simulink model "QR2Dsim"  (R2013b)
settings: Solver=ode3  StartTime=0.0  StopTime=Tend_sim  FixedStep=.01  RelTol=1e-3
values from neighbouring files (symbols this model uses):
  b = 0.1    [QR2Drunfile.m]
  ctauf = 8.004e-3    (= 0.008004)    [QR2Drunfile.m]
  d = 0.1    [QR2Drunfile.m]
  DeltaR = [0.2; -0.1; 0.02]    [QR2Drunfile.m]
  Deltax = [-0.5; 0.2; 1]    [QR2Drunfile.m]
  dxL0 = 0    [QR2Drunfile.m]
  dyL0 = 0    [QR2Drunfile.m]
  dzL0 = 0    [QR2Drunfile.m]
  e3 = [0;0;1]    [QR2Drunfile.m]
  fc = (mQ+mL)*g    (= 44.5374)    [QR2Drunfile.m]
  fsat = [-1000 1000]    [QR2Drunfile.m]
  g = 9.81    [QR2Drunfile.m]
  I = diag([Ixx Iyy Izz])    [QR2Drunfile.m]
  Ir = 0.5    [QR2Drunfile.m]
  Ixx = 0.0820    (= 0.082)    [QR2Drunfile.m]
  Iyy = 0    [QR2Drunfile.m]
  Izz = 0    [QR2Drunfile.m]
  kdL = 1.4    [QR2Drunfile.m]
  kdQ = 5.6*mQ*.75    (= 18.228)    [QR2Drunfile.m]
  kdxL = 1    [QR2Drunfile.m]
  kOmega = kOmega_phi*eye(3)    [QR2Drunfile.m]
  kpL = 1.2    [QR2Drunfile.m]
  kpQ = 16*mQ    (= 69.44)    [QR2Drunfile.m]
  kpxL = 5    [QR2Drunfile.m]
  kR = kR_phi*eye(3)    [QR2Drunfile.m]
  l = 0.315    [QR2Drunfile.m]
  lL = 0.4    [QR2Drunfile.m]
  mL = 0.2    [QR2Drunfile.m]
  mode = 2    [QR2Drunfile.m]
  mQ = 4.34    [QR2Drunfile.m]
  omega0 = [0;0;0]    [QR2Drunfile.m]
  phiL0 = deg2rad(190)    [QR2Drunfile.m]
  phiLd = 0    [QR2Drunfile.m]
  phiQ0 = deg2rad(0)    [QR2Drunfile.m]
  phiQd = 0    [QR2Drunfile.m]
  pL0 = 0    [QR2Drunfile.m]
  pQ0 = 0    [QR2Drunfile.m]
  psiL0 = 0    [QR2Drunfile.m]
  psiQ0 = 0    [QR2Drunfile.m]
  qL0 = 0    [QR2Drunfile.m]
  qQ0 = 0    [QR2Drunfile.m]
  qvec0 = [0; sin(phiL0); cos(phiL0)]    [QR2Drunfile.m]
  Rinit = Rx    [QR2Drunfile.m]
  rL0 = 0    [QR2Drunfile.m]
  rQ0 = 0    [QR2Drunfile.m]
  thetaL0 = 0    [QR2Drunfile.m]
  thetaQ0 = 0    [QR2Drunfile.m]
  xLd = [0; 0; 0]    [QR2Drunfile.m]
undefined symbols (not defined in the file or in its folder): dx0, dy0, dz0, kv, kx, m, p0, q0, r0, x0, y0, z0
libraries: simulink_extras x10, vrlib x9, dspmathops x2
(part 1 of 2)
settings Model: Creator=Nam  LastModifiedBy=Nam
settings DataIOCC: SaveFormat=StructureWithTime
settings DebuggingCC: SolverPrmCheckMsg=none

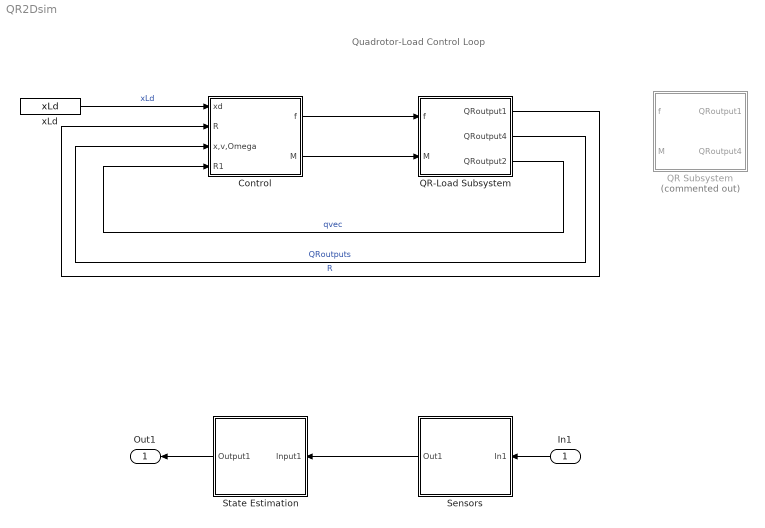
== system QR2Dsim ==
  note: Quadrotor-Load Control Loop
  In1 : Inport
  Control : Subsystem
  QR Subsystem : Subsystem  Commented=on
      mask Display: image('bebop.png')
  QR-Load Subsystem : Subsystem
  Sensors : Subsystem
      mask Display: image('optitrack.jpg')
  State Estimation : Subsystem
  xLd : Constant  Value=xLd  VectorParams1D=off
  Out1 : Outport
  wires:
  Sensors/1(Out1) -> State Estimation/1(Input1)
  State Estimation/1(Output1) -> Out1/1
  In1/1 -> Sensors/1(In1)
  QR-Load Subsystem/1(QRoutput1) -> Control/2(R)  "R"
  QR-Load Subsystem/2(QRoutput4) -> Control/3(x,v,Omega)  "QRoutputs"
  xLd/1 -> Control/1(xd)  "xLd"
  Control/1(f) -> QR-Load Subsystem/1(f)
  Control/2(M) -> QR-Load Subsystem/2(M)
  QR-Load Subsystem/3(QRoutput2) -> Control/4(R1)  "qvec"

== system QR2Dsim/Control ==
  note: Control
  xd : Inport
  R : Inport  Port=2
  x,v,Omega : Inport  Port=3
  R1 : Inport  Port=4
  QRL Load Attitude Controller : Subsystem
  QRL Load Position Controller : Subsystem
  QRL QR Attitude Controller : Subsystem
  Saturation : Saturate  UpperLimit=fsat(2)  LowerLimit=fsat(1)
  Terminator : Terminator
  f : Outport
  M : Outport  Port=2
  wires:
  R/1 -> QRL Load Position Controller/3(R1), QRL Load Attitude Controller/4(R), QRL QR Attitude Controller/3(R)
  x,v,Omega/1 -> QRL Load Attitude Controller/3(QROutput), QRL QR Attitude Controller/2(Omega), QRL Load Position Controller/2(QROutput1)
  Saturation/1 -> f/1  "f"
  xd/1 -> QRL Load Position Controller/1(xdes)
  QRL Load Position Controller/1(f) -> QRL Load Attitude Controller/1(xdes2), Saturation/1
  QRL QR Attitude Controller/1(M) -> M/1  "M"
  R1/1 -> Terminator/1  "qvec"
  QRL Load Attitude Controller/1(b3d1) -> QRL QR Attitude Controller/1(b1d)  "phiQc"
  QRL Load Position Controller/2(b3d1) -> QRL Load Attitude Controller/2(xdes1)

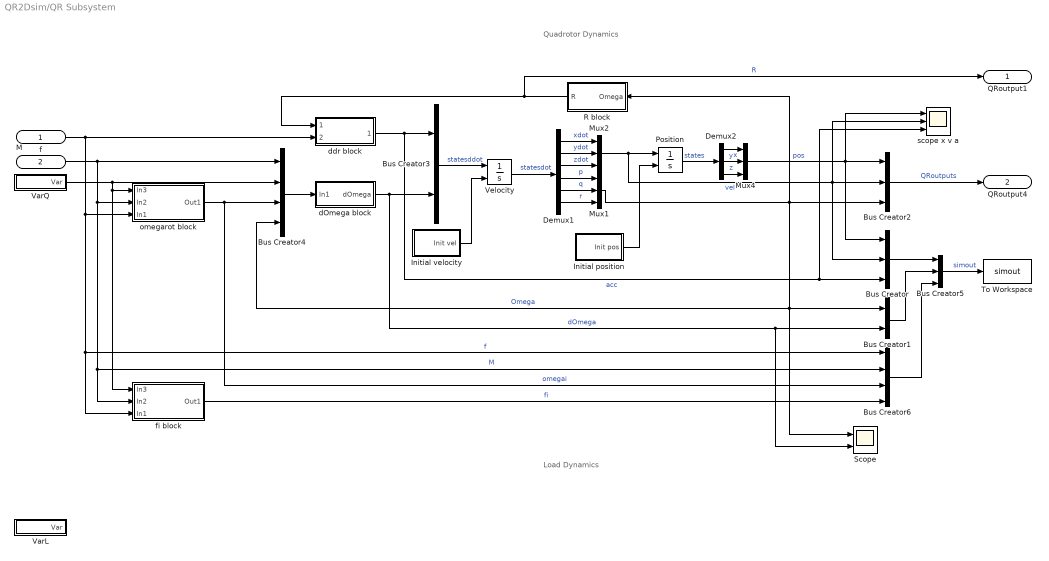
== system QR2Dsim/QR Subsystem ==
  note: Quadrotor Dynamics
  note: Load Dynamics
  f : Inport
  M : Inport  Port=2  PortDimensions=[3 1]
  Bus Creator : BusCreator  Inputs=3
  Bus Creator1 : BusCreator  Inputs=2
  Bus Creator2 : BusCreator  Inputs=3
  Bus Creator3 : BusCreator  Inputs=2
  Bus Creator4 : BusCreator
  Bus Creator5 : BusCreator  Inputs=3
  Bus Creator6 : BusCreator
  Demux1 : Demux  Outputs=6
  Demux2 : Demux  Outputs=3
  Initial position : Subsystem
  Initial velocity : Subsystem
  Mux1 : Mux  Inputs=3
  Mux2 : Mux  Inputs=3
  Mux4 : Mux  Inputs=3
  Position : Integrator  InitialConditionSource=external  ContinuousStateAttributes='position'
  R block : Subsystem
      mask Display: disp('R\prime = R \Omega_{\times}','texmode','on')
  Scope : Scope  NumInputPorts=2
      settings: ShowLegends=on  YMin=-5~-5  YMax=5~5  SaveName=ScopeData21
  To Workspace : ToWorkspace  VariableName=simout  SampleTime=-1  SaveFormat=Structure With Time
  VarL : Subsystem
  VarQ : Subsystem
  Velocity : Integrator  InitialConditionSource=external  ContinuousStateAttributes='velocity'
  dOmega block : Subsystem
      mask Display: disp('[p\prime; q\prime; r\prime]','texmode','on')
  ddr block : Subsystem
      mask Display: disp('[x\prime\prime; y\prime\prime; z\prime\prime]','texmode','on')
  fi block : Subsystem
      mask Display: disp('(f,M) \rightarrow f_i','texmode','on')
  omegarot block : Subsystem
      mask Display: disp('(f,M) \rightarrow \omega_i','texmode','on')
  scope x v a : Scope  NumInputPorts=3
      settings: ShowLegends=on  YMin=-10000~-500~0  YMax=180000~9000~225  SaveName=ScopeData12
  QRoutput1 : Outport
  QRoutput4 : Outport  Port=2
  wires:
  Velocity/1 -> Demux1/1  "statesdot"
  Position/1 -> Demux2/1  "states"
  ddr block/1(rddotOutput) -> Bus Creator3/1, Bus Creator/3, scope x v a/3  "acc"
  Bus Creator3/1 -> Velocity/1  "statesddot"
  dOmega block/1(dOmega) -> Bus Creator3/2, Bus Creator1/2, Scope/2  "dOmega"
  Bus Creator4/1 -> dOmega block/1(In1)
  Demux1/4 -> Mux1/1  "p"
  Demux1/5 -> Mux1/2  "q"
  Demux1/6 -> Mux1/3  "r"
  Demux1/2 -> Mux2/2  "ydot"
  Demux1/1 -> Mux2/1  "xdot"
  Demux1/3 -> Mux2/3  "zdot"
  Demux2/2 -> Mux4/2  "y"
  Demux2/1 -> Mux4/1  "x"
  Demux2/3 -> Mux4/3  "z"
  Mux4/1 -> scope x v a/1, Bus Creator/1, Bus Creator2/1  "pos"
  omegarot block/1(Out1) -> Bus Creator6/3, Bus Creator4/3  "omegai"
  Bus Creator/1 -> Bus Creator5/1
  Bus Creator1/1 -> Bus Creator5/2
  Bus Creator5/1 -> To Workspace/1  "simout"
  Mux1/1 -> Bus Creator2/3, R block/1(Omega), Bus Creator1/1, Scope/1, Bus Creator4/4  "Omega"
  Bus Creator2/1 -> QRoutput4/1  "QRoutputs"
  f/1 -> fi block/3(In1), Bus Creator6/1, omegarot block/3(In1), ddr block/2(R,f,m,g)  "f"
  VarQ/1(Var) -> fi block/1(In3), omegarot block/1(In3), Bus Creator4/2
  M/1 -> Bus Creator6/2, fi block/2(In2), omegarot block/2(In2), Bus Creator4/1  "M"
  Mux2/1 -> Position/1, scope x v a/2, Bus Creator/2, Bus Creator2/2  "vel"
  R block/1(R) -> ddr block/1(R,f,m,g1), QRoutput1/1  "R"
  Initial velocity/1(Init vel) -> Velocity/2
  Initial position/1(Init pos) -> Position/2
  fi block/1(Out1) -> Bus Creator6/4  "fi"
  Bus Creator6/1 -> Bus Creator5/3

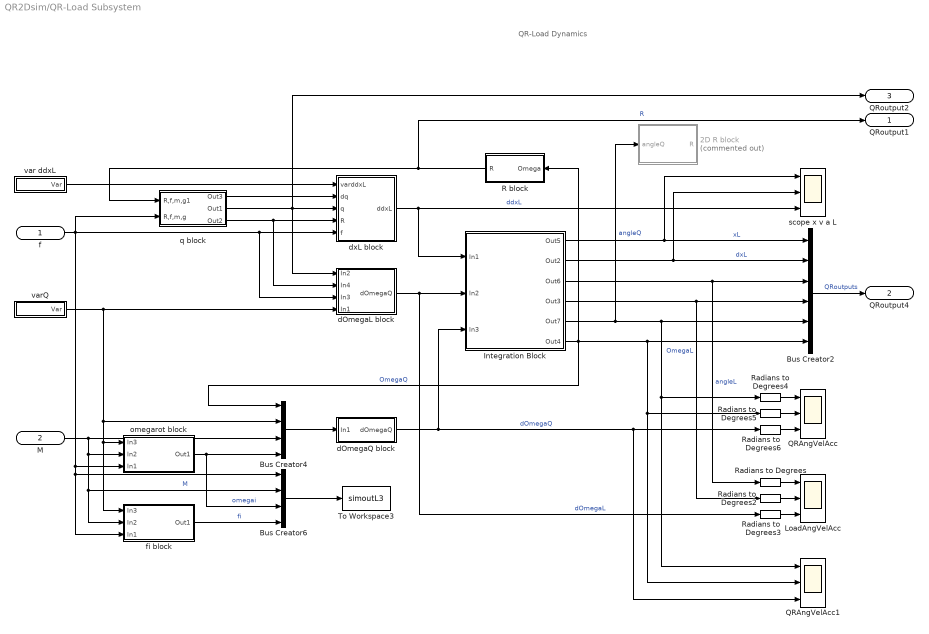
== system QR2Dsim/QR-Load Subsystem ==
  note: QR-Load Dynamics
  f : Inport
  M : Inport  Port=2  PortDimensions=3
  2D R block : MATLAB Function  Commented=on  TreatAsAtomicUnit=on
  Bus Creator2 : BusCreator  Inputs=6
  Bus Creator4 : BusCreator
  Bus Creator6 : BusCreator
  Integration Block : Subsystem
  LoadAngVelAcc : Scope  NumInputPorts=3
      settings: ShowLegends=on  YMin=-5~-5~-5  YMax=5~5~5  SaveName=ScopeData4
  QRAngVelAcc : Scope  NumInputPorts=3
      settings: ShowLegends=on  YMin=-5~-5~-5  YMax=5~5~5  SaveName=ScopeData3
  QRAngVelAcc1 : Scope  NumInputPorts=3
      settings: ShowLegends=on  YMin=-5~-5~-5  YMax=5~5~5  SaveName=ScopeData15
  R block : Subsystem
      mask Display: disp('R\prime = R \Omega_{\times}','texmode','on')
  Radians to Degrees{,2..6} (6 alike) : simulink_extras/Transformations/Radians to Degrees
  To Workspace3 : ToWorkspace  VariableName=simoutL3  SampleTime=-1  SaveFormat=Structure With Time
  dOmegaL block : Subsystem
  dOmegaQ block : Subsystem
  dxL block : MATLAB Function  TreatAsAtomicUnit=on
  fi block : Subsystem
      mask Display: disp('(f,M) \rightarrow f_i','texmode','on')
  omegarot block : Subsystem
      mask Display: disp('(f,M) \rightarrow \omega_i','texmode','on')
  q block : Subsystem
  scope x v a L : Scope  NumInputPorts=3
      settings: ShowLegends=on  YMin=-10000~-500~0  YMax=180000~9000~225  SaveName=ScopeData12
  var ddxL : Subsystem
  varQ : Subsystem
  QRoutput1 : Outport
  QRoutput4 : Outport  Port=2
  QRoutput2 : Outport  Port=3
  wires:
  dxL block/1(ddxL) -> scope x v a L/3, Integration Block/1(In1)  "ddxL"
  dOmegaQ block/1(dOmegaQ) -> Integration Block/3(In3), Radians to Degrees6/1, QRAngVelAcc1/3  "dOmegaQ"
  Bus Creator4/1 -> dOmegaQ block/1(In1)
  omegarot block/1(Out1) -> Bus Creator6/3, Bus Creator4/4  "omegai"
  Bus Creator2/1 -> QRoutput4/1  "QRoutputs"
  f/1 -> q block/2(R,f,m,g), dxL block/5(f), dOmegaL block/3(In3), omegarot block/3(In1), Bus Creator6/1, fi block/3(In1)
  M/1 -> fi block/2(In2), Bus Creator6/2, omegarot block/2(In2), Bus Creator4/3  "M"
  fi block/1(Out1) -> Bus Creator6/4  "fi"
  var ddxL/1(Var) -> dxL block/1(varddxL)
  q block/2(Out1) -> dxL block/3(q), QRoutput2/1, dOmegaL block/1(In2)
  q block/3(Out2) -> dxL block/4(R), dOmegaL block/2(In4)
  q block/1(Out3) -> dxL block/2(dq)
  Integration Block/5(Out7) -> Radians to Degrees4/1, QRAngVelAcc1/1, Bus Creator2/5, 2D R block/1(angleQ)  "angleQ"
  Integration Block/2(Out2) -> scope x v a L/2, Bus Creator2/2  "dxL"
  Integration Block/4(Out3) -> Bus Creator2/4, Radians to Degrees2/1  "OmegaL"
  Integration Block/6(Out4) -> R block/1(Omega), Radians to Degrees5/1, QRAngVelAcc1/2, Bus Creator2/6, Bus Creator4/1  "OmegaQ"
  Integration Block/1(Out5) -> scope x v a L/1, Bus Creator2/1  "xL"
  dOmegaL block/1(dOmegaQ) -> Radians to Degrees3/1, Integration Block/2(In2)  "dOmegaL"
  varQ/1(Var) -> Bus Creator4/2, fi block/1(In3), omegarot block/1(In3), dOmegaL block/4(In1)
  Integration Block/3(Out6) -> Bus Creator2/3, Radians to Degrees/1  "angleL"
  Bus Creator6/1 -> To Workspace3/1
  Radians to Degrees/1 -> LoadAngVelAcc/1
  Radians to Degrees2/1 -> LoadAngVelAcc/2
  Radians to Degrees3/1 -> LoadAngVelAcc/3
  Radians to Degrees5/1 -> QRAngVelAcc/2
  Radians to Degrees4/1 -> QRAngVelAcc/1
  Radians to Degrees6/1 -> QRAngVelAcc/3
  R block/1(R) -> q block/1(R,f,m,g1), QRoutput1/1  "R"

== system QR2Dsim/Sensors ==
  In1 : Inport
  Out1 : Outport
  wires:
  In1/1 -> Out1/1

== system QR2Dsim/State Estimation ==
  Input1 : Inport
  Output1 : Outport
  wires:
  Input1/1 -> Output1/1

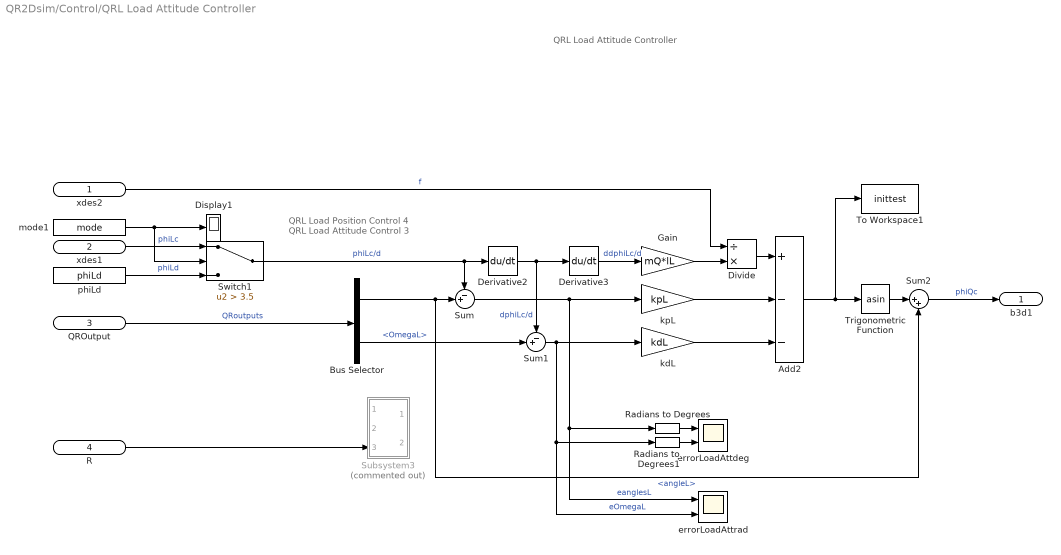
== system QR2Dsim/Control/QRL Load Attitude Controller ==
  note: QRL Load Attitude Controller
  note: QRL Load Position Control 4
      | QRL Load Attitude Control 3
  xdes2 : Inport
  xdes1 : Inport  Port=2
  QROutput : Inport  Port=3
  R : Inport  Port=4
  Add2 : Sum  Inputs=+--
  Bus Selector : BusSelector  OutputSignals=angleL,OmegaL
  Derivative2 : Derivative
  Derivative3 : Derivative
  Display1 : Display
  Divide : Product  Inputs=/*
  Gain : Gain  Gain=mQ*lL
  Radians to Degrees : simulink_extras/Transformations/Radians to Degrees
  Radians to Degrees1 : simulink_extras/Transformations/Radians to Degrees
  Subsystem3 : Subsystem  Commented=on
  Sum : Sum  Inputs=-+|
  Sum1 : Sum  Inputs=-+|
  Sum2 : Sum  Inputs=|++
  Switch1 : Switch  Criteria=u2 > Threshold  Threshold=3.5
  To Workspace1 : ToWorkspace  VariableName=inittest  SampleTime=-1  SaveFormat=Structure With Time
  Trigonometric Function : Trigonometry  Operator=asin
  errorLoadAttdeg : Scope  NumInputPorts=2
      settings: YMin=-5~-5  YMax=5~5  SaveName=ScopeData14
  errorLoadAttrad : Scope  NumInputPorts=2
      settings: YMin=-5~-5  YMax=5~5  SaveName=ScopeData26
  kdL : Gain  Gain=kdL
  kpL : Gain  Gain=kpL
  mode1 : Constant  Value=mode  VectorParams1D=off
  phiLd : Constant  Value=phiLd  VectorParams1D=off
  b3d1 : Outport
  wires:
  QROutput/1 -> Bus Selector/1  "QRoutputs"
  Sum/1 -> kpL/1, errorLoadAttrad/1, Radians to Degrees/1  "eanglesL"
  Sum1/1 -> kdL/1, errorLoadAttrad/2, Radians to Degrees1/1  "eOmegaL"
  kpL/1 -> Add2/2
  kdL/1 -> Add2/3
  Derivative2/1 -> Sum1/1, Derivative3/1  "dphiLc/d"
  Derivative3/1 -> Gain/1  "ddphiLc/d"
  Bus Selector/1 -> Sum2/2, Sum/2  "<angleL>"
  Bus Selector/2 -> Sum1/2  "<OmegaL>"
  Switch1/1 -> Derivative2/1, Sum/1  "phiLc/d"
  xdes1/1 -> Switch1/1  "phiLc"
  phiLd/1 -> Switch1/3  "phiLd"
  Sum2/1 -> b3d1/1  "phiQc"
  Gain/1 -> Divide/2
  Divide/1 -> Add2/1
  Add2/1 -> To Workspace1/1, Trigonometric Function/1
  Trigonometric Function/1 -> Sum2/1
  R/1 -> Subsystem3/3(In3)
  Radians to Degrees/1 -> errorLoadAttdeg/1
  Radians to Degrees1/1 -> errorLoadAttdeg/2
  xdes2/1 -> Divide/1  "f"
  mode1/1 -> Switch1/2, Display1/1

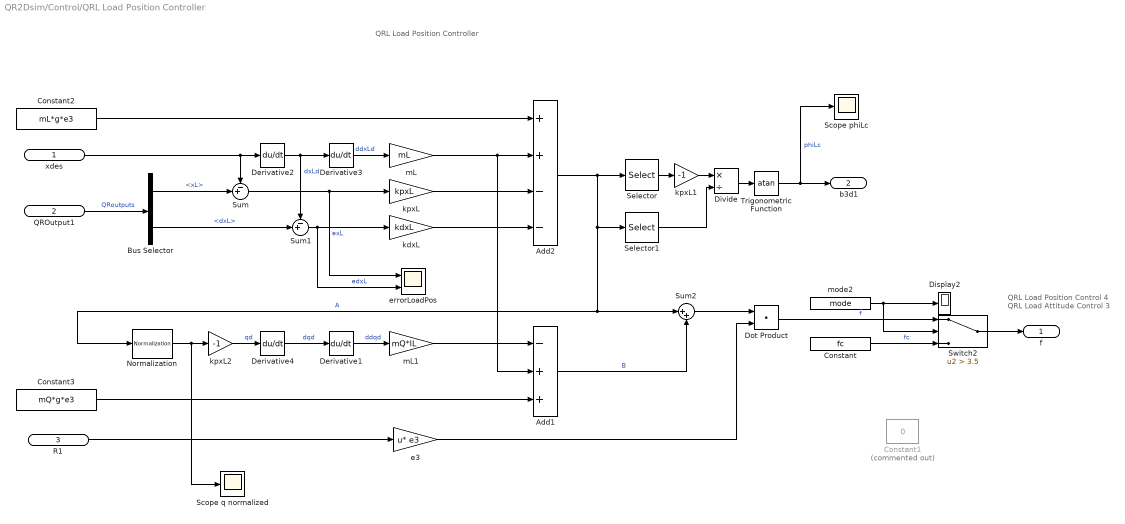
== system QR2Dsim/Control/QRL Load Position Controller ==
  note: QRL Load Position Controller
  note: QRL Load Position Control 4
      | QRL Load Attitude Control 3
  xdes : Inport
  QROutput1 : Inport  Port=2
  R1 : Inport  Port=3
  Add1 : Sum  Inputs=-++
  Add2 : Sum  Inputs=++--
  Bus Selector : BusSelector  OutputSignals=xL,dxL
  Constant : Constant  Value=fc
  Constant1 : Constant  Commented=on  Value=0
  Constant2 : Constant  Value=mL*g*e3
  Constant3 : Constant  Value=mQ*g*e3
  Derivative{1..4} (4 alike) : Derivative
  Display2 : Display
  Divide : Product  Inputs=*/
  Dot Product : DotProduct  InputSameDT=on  OutDataTypeStr=Inherit: Inherit via internal rule
  Normalization : dspmathops/Normalization  NormType=2-norm  Bias=1e-10  NormOver=Each column  ColComp=on  Dimension=1  outputDataTypeStr=Inherit: Same as product output  outputLastDataTypeStr=Inherit: Same as product output  outputMin=[]  outputMax=[]  accumDataTypeStr=Inherit: Same as product output  accumLastDataTypeStr=Inherit: Same as product output  roundingMode=Floor  overflowMode=off
  Scope phiLc : Scope
      settings: SaveName=ScopeData27
  Scope q normalized : Scope
      settings: SaveName=ScopeData29
  Selector : Selector  InputPortWidth=3  IndexOptions=Index vector (dialog)  Indices=2  OutputSizes=1
  Selector1 : Selector  InputPortWidth=3  IndexOptions=Index vector (dialog)  Indices=3  OutputSizes=1
  Sum : Sum  Inputs=-+|
  Sum1 : Sum  Inputs=-+|
  Sum2 : Sum  Inputs=|++
  Switch2 : Switch  Criteria=u2 > Threshold  Threshold=3.5
  Trigonometric Function : Trigonometry  Operator=atan
  e3 : Gain  Gain=e3  Multiplication=Matrix(u*K)
  errorLoadPos : Scope  NumInputPorts=2
      settings: YMin=-5~-5  YMax=5~5  SaveName=ScopeData28
  kdxL : Gain  Gain=kdxL
  kpxL : Gain  Gain=kpxL
  kpxL1 : Gain  Gain=-1
  kpxL2 : Gain  Gain=-1
  mL : Gain  Gain=mL
  mL1 : Gain  Gain=mQ*lL
  mode2 : Constant  Value=mode  VectorParams1D=off
  f : Outport
  b3d1 : Outport  Port=2
  wires:
  QROutput1/1 -> Bus Selector/1  "QRoutputs"
  Sum/1 -> kpxL/1, errorLoadPos/1  "exL"
  Sum1/1 -> kdxL/1, errorLoadPos/2  "edxL"
  kpxL/1 -> Add2/3
  kdxL/1 -> Add2/4
  Derivative2/1 -> Sum1/1, Derivative3/1  "dxLd"
  Derivative3/1 -> mL/1  "ddxLd"
  Bus Selector/1 -> Sum/2  "<xL>"
  Bus Selector/2 -> Sum1/2  "<dxL>"
  xdes/1 -> Derivative2/1, Sum/1
  mL/1 -> Add1/2, Add2/2
  Constant2/1 -> Add2/1
  Add2/1 -> Normalization/1, Sum2/1, Selector1/1, Selector/1  "A"
  R1/1 -> e3/1
  e3/1 -> Dot Product/2
  Add1/1 -> Sum2/2  "B"
  Sum2/1 -> Dot Product/1
  Selector/1 -> kpxL1/1
  kpxL1/1 -> Divide/1
  Selector1/1 -> Divide/2
  Divide/1 -> Trigonometric Function/1
  Trigonometric Function/1 -> Scope phiLc/1, b3d1/1  "phiLc"
  Normalization/1 -> Scope q normalized/1, kpxL2/1
  kpxL2/1 -> Derivative4/1  "qd"
  Derivative4/1 -> Derivative1/1  "dqd"
  Derivative1/1 -> mL1/1  "ddqd"
  mL1/1 -> Add1/1
  Constant3/1 -> Add1/3
  Constant/1 -> Switch2/3  "fc"
  mode2/1 -> Switch2/2, Display2/1
  Switch2/1 -> f/1
  Dot Product/1 -> Switch2/1  "f"

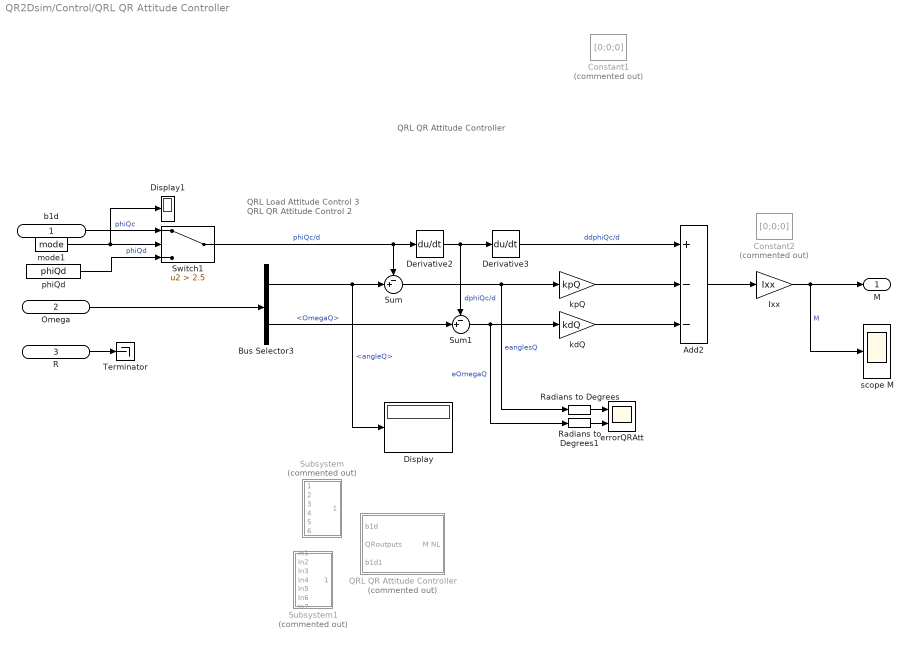
== system QR2Dsim/Control/QRL QR Attitude Controller ==
  note: QRL QR Attitude Controller
  note: QRL Load Attitude Control 3
      | QRL QR Attitude Control 2
  b1d : Inport
  Omega : Inport  Port=2
  R : Inport  Port=3
  Add2 : Sum  Inputs=+--
  Bus Selector3 : BusSelector  OutputSignals=angleQ,OmegaQ
  Constant1 : Constant  Commented=on  Value=[0;0;0]
  Constant2 : Constant  Commented=on  Value=[0;0;0]
  Derivative2 : Derivative
  Derivative3 : Derivative
  Display : Display
  Display1 : Display
  Ixx : Gain  Gain=Ixx
  QRL QR Attitude Controller : Subsystem  Commented=on
  Radians to Degrees : simulink_extras/Transformations/Radians to Degrees
  Radians to Degrees1 : simulink_extras/Transformations/Radians to Degrees
  Subsystem : Subsystem  Commented=on
  Subsystem1 : Subsystem  Commented=on
  Sum : Sum  Inputs=-+|
  Sum1 : Sum  Inputs=-+|
  Switch1 : Switch  Criteria=u2 > Threshold  Threshold=2.5
  Terminator : Terminator
  errorQRAtt : Scope  NumInputPorts=2
      settings: YMin=-5~-5  YMax=5~5  SaveName=ScopeData6
  kdQ : Gain  Gain=kdQ
  kpQ : Gain  Gain=kpQ
  mode1 : Constant  Value=mode  VectorParams1D=off
  phiQd : Constant  Value=phiQd  VectorParams1D=off
  scope M : Scope
      settings: ShowLegends=on  SaveName=ScopeData19
  M : Outport  PortDimensions=3
  wires:
  mode1/1 -> Display1/1, Switch1/2
  b1d/1 -> Switch1/1  "phiQc"
  phiQd/1 -> Switch1/3  "phiQd"
  Omega/1 -> Bus Selector3/1
  Sum/1 -> Radians to Degrees/1, kpQ/1  "eanglesQ"
  Sum1/1 -> Radians to Degrees1/1, kdQ/1  "eOmegaQ"
  Ixx/1 -> scope M/1, M/1  "M"
  kpQ/1 -> Add2/2
  kdQ/1 -> Add2/3
  Add2/1 -> Ixx/1
  Switch1/1 -> Derivative2/1, Sum/1  "phiQc/d"
  Derivative2/1 -> Sum1/1, Derivative3/1  "dphiQc/d"
  Derivative3/1 -> Add2/1  "ddphiQc/d"
  Bus Selector3/1 -> Sum/2, Display/1  "<angleQ>"
  Bus Selector3/2 -> Sum1/2  "<OmegaQ>"
  R/1 -> Terminator/1
  Radians to Degrees/1 -> errorQRAtt/1
  Radians to Degrees1/1 -> errorQRAtt/2

== system QR2Dsim/QR Subsystem/Initial position ==
  Bus Creator2 : BusCreator  Inputs=3
  x0 : Constant  Value=x0
  y0 : Constant  Value=y0
  z0 : Constant  Value=z0
  Init pos : Outport
  wires:
  y0/1 -> Bus Creator2/2  "y0"
  x0/1 -> Bus Creator2/1  "x0"
  z0/1 -> Bus Creator2/3  "z0"
  Bus Creator2/1 -> Init pos/1  "Init pos"

== system QR2Dsim/QR Subsystem/Initial velocity ==
  Bus Creator1 : BusCreator  Inputs=6
  dx0 : Constant  Value=dx0
  dy0 : Constant  Value=dy0
  dz0 : Constant  Value=dz0
  p0 : Constant  Value=p0
  q0 : Constant  Value=q0
  r0 : Constant  Value=r0
  Init vel : Outport
  wires:
  p0/1 -> Bus Creator1/4  "p0"
  dx0/1 -> Bus Creator1/1  "dx0"
  dz0/1 -> Bus Creator1/3  "dz0"
  dy0/1 -> Bus Creator1/2  "dy0"
  q0/1 -> Bus Creator1/5  "q0"
  r0/1 -> Bus Creator1/6  "r0"
  Bus Creator1/1 -> Init vel/1  "Init vel"

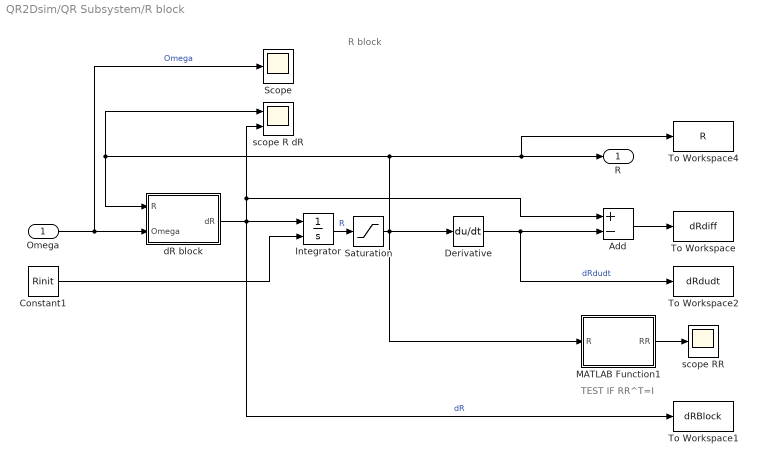
== system QR2Dsim/QR Subsystem/R block ==
  note: R block
  note: TEST IF RR^T=I
  Omega : Inport
  Add : Sum  Inputs=+-
  Constant1 : Constant  Value=Rinit
  Derivative : Derivative
  Integrator : Integrator  InitialConditionSource=external  ContinuousStateAttributes='R'
  MATLAB Function1 : MATLAB Function  TreatAsAtomicUnit=on
  Saturation : Saturate  UpperLimit=1  LowerLimit=-1
  Scope : Scope
      settings: ShowLegends=on  SaveName=ScopeData9
  To Workspace : ToWorkspace  VariableName=dRdiff  SampleTime=-1  SaveFormat=Structure With Time
  To Workspace1 : ToWorkspace  VariableName=dRBlock  SampleTime=-1  SaveFormat=Structure With Time
  To Workspace2 : ToWorkspace  VariableName=dRdudt  SampleTime=-1  SaveFormat=Structure With Time
  To Workspace4 : ToWorkspace  VariableName=R  SampleTime=-1  SaveFormat=Structure With Time
  dR block : MATLAB Function  TreatAsAtomicUnit=on
  scope R dR : Scope  NumInputPorts=2
      settings: ShowLegends=on  YMin=-1.2~-4e+19  YMax=1.2~4e+19  SaveName=ScopeData16
  scope RR : Scope
      settings: SaveName=ScopeData17
  R : Outport
  wires:
  Integrator/1 -> Saturation/1  "R"
  dR block/1(dR) -> scope R dR/2, Add/1, To Workspace1/1, Integrator/1  "dR"
  Omega/1 -> Scope/1, dR block/2(Omega)  "Omega"
  Derivative/1 -> Add/2, To Workspace2/1  "dRdudt"
  Add/1 -> To Workspace/1
  MATLAB Function1/1(RR) -> scope RR/1
  Constant1/1 -> Integrator/2
  Saturation/1 -> MATLAB Function1/1(R), Derivative/1, dR block/1(R), scope R dR/1, R/1, To Workspace4/1

== system QR2Dsim/QR Subsystem/VarL ==
  Bus Creator : BusCreator  Inputs=2
  Bus Creator1 : BusCreator  Inputs=2
  Cable length : Constant  Value=lL
  Gravity Constant : Constant  Value=g
  Mass Load : Constant  Value=mL
  Var : Outport
  wires:
  Gravity Constant/1 -> Bus Creator/2  "g"
  Bus Creator/1 -> Var/1  "varL"
  Mass Load/1 -> Bus Creator1/1  "mL"
  Cable length/1 -> Bus Creator1/2  "lL"
  Bus Creator1/1 -> Bus Creator/1  "sysvar"

== system QR2Dsim/QR Subsystem/VarQ ==
  Arm length : Constant  Value=l
  Bus Creator : BusCreator  Inputs=2
  Bus Creator1 : BusCreator  Inputs=7
  Drag Factor : Constant  Value=d
  Gravity Constant : Constant  Value=g
  Mass QR : Constant  Value=mQ
  QR Inertia : Constant  Value=diag([Ixx,Iyy,Izz])
  Rotor Inertia : Constant  Value=Ir
  Thrust Factor : Constant  Value=b
  ctauf : Constant  Value=ctauf
      mask Display: disp('c_{\tau f}','texmode','on')
  Var : Outport
  wires:
  Gravity Constant/1 -> Bus Creator/2  "g"
  Bus Creator/1 -> Var/1  "varQ"
  Mass QR/1 -> Bus Creator1/1  "m"
  Arm length/1 -> Bus Creator1/6  "l"
  Rotor Inertia/1 -> Bus Creator1/5  "Ir"
  QR Inertia/1 -> Bus Creator1/2  "I"
  Bus Creator1/1 -> Bus Creator/1  "sysvar"
  Thrust Factor/1 -> Bus Creator1/3  "b"
  Drag Factor/1 -> Bus Creator1/4  "d"
  ctauf/1 -> Bus Creator1/7  "ctauf"

== system QR2Dsim/QR Subsystem/dOmega block ==
  In1 : Inport
  Add : Sum  Inputs=-+
  Bus Selector : BusSelector  OutputSignals=Omega,varQ.sysvar.Ir,omegai,M
  DeltaR : Constant  Value=DeltaR
      mask Display: disp('\Delta_R','texmode','on')
  Gain : Gain  Gain=inv(I)  Multiplication=Matrix(K*u)
  Subsystem1 : Subsystem
      mask Display: disp('\Omega \times I\Omega','texmode','on')
  Subsystem2 : Subsystem
      mask Display: disp('\tau_G=\Sigma I_R(\omega \times e_3) \omega_i ','texmode','on')
  Terminator : Terminator
  Terminator1 : Terminator
  dOmega : Outport
  wires:
  In1/1 -> Bus Selector/1
  Bus Selector/1 -> Subsystem1/1(Omega), Subsystem2/1(In1)  "<Omega>"
  Bus Selector/2 -> Subsystem2/2(In2)  "<Ir>"
  Bus Selector/4 -> Add/2  "<M>"
  Subsystem2/1(Out1) -> Terminator/1
  Bus Selector/3 -> Subsystem2/3(In3)  "<omegai>"
  DeltaR/1 -> Terminator1/1  "DeltaR"
  Subsystem1/1(Out1) -> Add/1
  Add/1 -> Gain/1  "J*dOmega"
  Gain/1 -> dOmega/1

== system QR2Dsim/QR Subsystem/ddr block ==
  R,f,m,g1 : Inport
  R,f,m,g : Inport  Port=2
  Deltax : Constant  Value=Deltax
      mask Display: disp('\Delta_x','texmode','on')
  Gain : Gain  Gain=e3  Multiplication=Matrix(u*K)
  Gain1 : Gain  Gain=1/m
  Product : Product
  Sum : Sum  Inputs=|-+
  Terminator : Terminator
  mge3 : Constant  Value=m*g*e3
  rddotOutput : Outport
  wires:
  R,f,m,g1/1 -> Gain/1  "R"
  R,f,m,g/1 -> Product/2  "f"
  Gain/1 -> Product/1
  Product/1 -> Sum/1
  mge3/1 -> Sum/2  "m"
  Sum/1 -> Gain1/1
  Gain1/1 -> rddotOutput/1  "a"
  Deltax/1 -> Terminator/1  "Deltax"

== system QR2Dsim/QR Subsystem/fi block ==
  In3 : Inport
  In2 : Inport  Port=2
  In1 : Inport  Port=3
  Bus Selector2 : BusSelector  OutputSignals=sysvar.l,sysvar.ctauf  OutputAsBus=on
  Saturation : Saturate  UpperLimit=inf  LowerLimit=-inf  ZeroCross=off
  fcnf : MATLAB Function  TreatAsAtomicUnit=on
  Out1 : Outport
  wires:
  In3/1 -> Bus Selector2/1
  In1/1 -> fcnf/3(f)  "f"
  In2/1 -> fcnf/2(M)  "M"
  Bus Selector2/1 -> fcnf/1(var)  "var"
  fcnf/1(fi) -> Saturation/1
  Saturation/1 -> Out1/1  "fi"

== system QR2Dsim/QR Subsystem/omegarot block ==
  In3 : Inport
  In2 : Inport  Port=2
  In1 : Inport  Port=3
  Bus Selector2 : BusSelector  OutputSignals=sysvar.b,sysvar.d,sysvar.l  OutputAsBus=on
  Saturation : Saturate  UpperLimit=inf  LowerLimit=0  ZeroCross=off
  Sqrt : Sqrt  SaturateOnIntegerOverflow=on
  fcnomega : MATLAB Function  TreatAsAtomicUnit=on
  Out1 : Outport
  wires:
  In3/1 -> Bus Selector2/1
  In1/1 -> fcnomega/3(f)  "f"
  In2/1 -> fcnomega/2(M)  "M"
  Bus Selector2/1 -> fcnomega/1(var)  "var"
  Sqrt/1 -> Out1/1  "omegai"
  Saturation/1 -> Sqrt/1
  fcnomega/1(omegai) -> Saturation/1  "omegai^2"

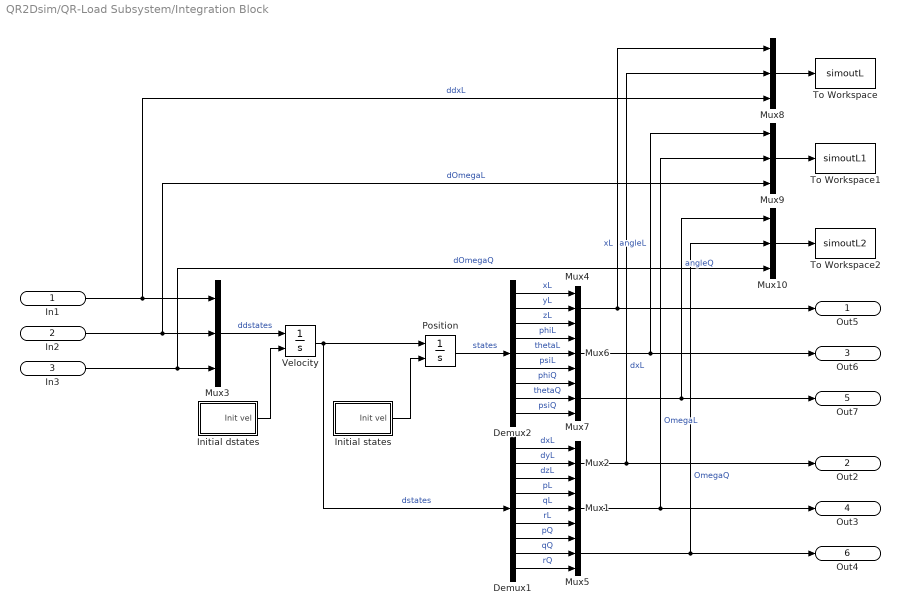
== system QR2Dsim/QR-Load Subsystem/Integration Block ==
  In1 : Inport
  In2 : Inport  Port=2
  In3 : Inport  Port=3
  Demux1 : Demux  Outputs=9
  Demux2 : Demux  Outputs=9
  Initial dstates : Subsystem
  Initial states : Subsystem
  Mux{1..10} (10 alike) : Mux  Inputs=3
  Position : Integrator  InitialConditionSource=external  ContinuousStateAttributes='position'
  To Workspace : ToWorkspace  VariableName=simoutL  SampleTime=-1  SaveFormat=Structure With Time
  To Workspace1 : ToWorkspace  VariableName=simoutL1  SampleTime=-1  SaveFormat=Structure With Time
  To Workspace2 : ToWorkspace  VariableName=simoutL2  SampleTime=-1  SaveFormat=Structure With Time
  Velocity : Integrator  InitialConditionSource=external  ContinuousStateAttributes='velocity'
  Out5 : Outport
  Out2 : Outport  Port=2
  Out6 : Outport  Port=3
  Out3 : Outport  Port=4
  Out7 : Outport  Port=5
  Out4 : Outport  Port=6
  wires:
  In1/1 -> Mux8/3, Mux3/1  "ddxL"
  Demux1/4 -> Mux1/1  "pL"
  Demux1/5 -> Mux1/2  "qL"
  Demux1/6 -> Mux1/3  "rL"
  Demux1/2 -> Mux2/2  "dyL"
  Demux1/1 -> Mux2/1  "dxL"
  Demux1/3 -> Mux2/3  "dzL"
  Demux1/8 -> Mux5/2  "qQ"
  Demux1/9 -> Mux5/3  "rQ"
  Demux1/7 -> Mux5/1  "pQ"
  Mux3/1 -> Velocity/1  "ddstates"
  Initial dstates/1(Init vel) -> Velocity/2
  Position/1 -> Demux2/1  "states"
  Demux2/2 -> Mux4/2  "yL"
  Demux2/1 -> Mux4/1  "xL"
  Demux2/3 -> Mux4/3  "zL"
  Initial states/1(Init vel) -> Position/2
  Demux2/4 -> Mux6/1  "phiL"
  Demux2/5 -> Mux6/2  "thetaL"
  Demux2/6 -> Mux6/3  "psiL"
  Demux2/9 -> Mux7/3  "psiQ"
  Demux2/8 -> Mux7/2  "thetaQ"
  Demux2/7 -> Mux7/1  "phiQ"
  Velocity/1 -> Position/1, Demux1/1  "dstates"
  Mux2/1 -> Mux8/2, Out2/1  "dxL"
  Mux4/1 -> Mux8/1, Out5/1  "xL"
  Mux1/1 -> Mux9/2, Out3/1  "OmegaL"
  In2/1 -> Mux9/3, Mux3/2  "dOmegaL"
  Mux6/1 -> Mux9/1, Out6/1  "angleL"
  In3/1 -> Mux10/3, Mux3/3  "dOmegaQ"
  Mux7/1 -> Mux10/1, Out7/1  "angleQ"
  Mux5/1 -> Mux10/2, Out4/1  "OmegaQ"
  Mux8/1 -> To Workspace/1
  Mux9/1 -> To Workspace1/1
  Mux10/1 -> To Workspace2/1

== system QR2Dsim/QR-Load Subsystem/R block ==
  note: R block
  Omega : Inport
  Constant1 : Constant  Value=Rinit
  Integrator : Integrator  InitialConditionSource=external  ContinuousStateAttributes='R'
  Saturation : Saturate  UpperLimit=1  LowerLimit=-1
  To Workspace4 : ToWorkspace  VariableName=R  SampleTime=-1  SaveFormat=Structure With Time
  dR block : MATLAB Function  TreatAsAtomicUnit=on
  R : Outport
  wires:
  Integrator/1 -> Saturation/1  "R"
  dR block/1(dR) -> Integrator/1
  Omega/1 -> dR block/2(Omega)
  Constant1/1 -> Integrator/2
  Saturation/1 -> dR block/1(R), To Workspace4/1, R/1  "R"

== system QR2Dsim/QR-Load Subsystem/dOmegaL block ==
  note: dOmegaL block
  In2 : Inport
  In4 : Inport  Port=2
  In3 : Inport  Port=3
  In1 : Inport  Port=4
  Bus Selector : BusSelector  OutputSignals=sysvar.m,sysvar.lL
  Cross Product : vrlib/Utilities/Cross Product
  Divide : Product  Inputs=*/
  Gain : Gain  Gain=-1
  Gain1 : Gain  Gain=e3  Multiplication=Matrix(u*K)
  Product1 : Product
  Product2 : Product
  dOmegaQ : Outport
  wires:
  In2/1 -> Gain/1  "q"
  In3/1 -> Product1/1  "f"
  In4/1 -> Gain1/1  "R"
  Gain/1 -> Cross Product/1
  Gain1/1 -> Product1/2  "Re3"
  Product1/1 -> Cross Product/2
  In1/1 -> Bus Selector/1  "varQ"
  Bus Selector/1 -> Product2/1  "<m>"
  Bus Selector/2 -> Product2/2  "<lL>"
  Cross Product/1 -> Divide/1
  Product2/1 -> Divide/2
  Divide/1 -> dOmegaQ/1  "dOmegaL"

== system QR2Dsim/QR-Load Subsystem/dOmegaQ block ==
  In1 : Inport
  Add : Sum  Inputs=-+
  Bus Selector : BusSelector  OutputSignals=OmegaQ,varQ.sysvar.Ir,omegai,M
  Gain1 : Gain  Gain=0
  Gain2 : Gain  Gain=inv(Ixx)
  Subsystem1 : Subsystem
      mask Display: disp('\Omega \times I\Omega','texmode','on')
  Subsystem2 : Subsystem
      mask Display: disp('\tau_G=\Sigma I_R(\omega \times e_3) \omega_i ','texmode','on')
  Terminator : Terminator
  dOmegaQ : Outport
  wires:
  In1/1 -> Bus Selector/1  "varQ"
  Bus Selector/1 -> Subsystem1/1(Omega), Subsystem2/1(In1)  "<OmegaQ>"
  Bus Selector/2 -> Subsystem2/2(In2)  "<Ir>"
  Subsystem2/1(Out1) -> Terminator/1
  Bus Selector/3 -> Subsystem2/3(In3)  "<omegai>"
  Subsystem1/1(Out1) -> Gain1/1
  Gain1/1 -> Add/1
  Add/1 -> Gain2/1  "J*dOmega"
  Bus Selector/4 -> Add/2  "<M>"
  Gain2/1 -> dOmegaQ/1  "dOmegaQ"

== system QR2Dsim/QR-Load Subsystem/fi block ==
  In3 : Inport
  In2 : Inport  Port=2
  In1 : Inport  Port=3
  Bus Selector2 : BusSelector  OutputSignals=sysvar.l,sysvar.ctauf  OutputAsBus=on
  Saturation : Saturate  UpperLimit=inf  LowerLimit=-inf  ZeroCross=off
  fcnf : MATLAB Function  TreatAsAtomicUnit=on
  Out1 : Outport
  wires:
  In3/1 -> Bus Selector2/1
  In1/1 -> fcnf/3(f)  "f"
  In2/1 -> fcnf/2(M)  "M"
  Bus Selector2/1 -> fcnf/1(var)  "var"
  fcnf/1(fi) -> Saturation/1
  Saturation/1 -> Out1/1  "fi"

== system QR2Dsim/QR-Load Subsystem/omegarot block ==
  In3 : Inport
  In2 : Inport  Port=2
  In1 : Inport  Port=3
  Bus Selector2 : BusSelector  OutputSignals=sysvar.b,sysvar.d,sysvar.l  OutputAsBus=on
  Saturation : Saturate  UpperLimit=inf  LowerLimit=0  ZeroCross=off
  Sqrt : Sqrt  SaturateOnIntegerOverflow=on
  fcnomega : MATLAB Function  TreatAsAtomicUnit=on
  Out1 : Outport
  wires:
  In3/1 -> Bus Selector2/1
  In1/1 -> fcnomega/3(f)  "f"
  In2/1 -> fcnomega/2(M)  "M"
  Bus Selector2/1 -> fcnomega/1(var)  "var"
  Sqrt/1 -> Out1/1  "omegai"
  Saturation/1 -> Sqrt/1
  fcnomega/1(omegai) -> Saturation/1  "omegai^2"

== system QR2Dsim/QR-Load Subsystem/q block ==
  note: q Block
  R,f,m,g1 : Inport
  R,f,m,g : Inport  Port=2
  1/(mQ*lL) : Gain  Gain=1/(mQ*lL)
  Cross Product : vrlib/Utilities/Cross Product
  Cross Product1 : vrlib/Utilities/Cross Product
  Gain : Gain  Gain=e3  Multiplication=Matrix(u*K)
  Gain1 : Gain  Gain=-1
  Integrator1 : Integrator  InitialCondition=qvec0  ContinuousStateAttributes='velocity'
  Integrator2 : Integrator  InitialCondition=omega0  ContinuousStateAttributes='velocity'
  Product : Product
  To Workspace1 : ToWorkspace  VariableName=qvec  SampleTime=-1  SaveFormat=Structure With Time
  Out3 : Outport
  Out1 : Outport  Port=2
  Out2 : Outport  Port=3
  wires:
  Cross Product/1 -> Integrator1/1, Out3/1  "dq"
  Integrator1/1 -> Out1/1, To Workspace1/1, Cross Product/2, Gain1/1  "q"
  Integrator2/1 -> Cross Product/1  "omega"
  R,f,m,g1/1 -> Gain/1, Out2/1  "R"
  Gain/1 -> Product/2  "Re3"
  Product/1 -> Cross Product1/2
  Gain1/1 -> Cross Product1/1
  Cross Product1/1 -> 1/(mQ*lL)/1
  1/(mQ*lL)/1 -> Integrator2/1  "domega"
  R,f,m,g/1 -> Product/1  "f"

== system QR2Dsim/QR-Load Subsystem/var ddxL ==
  Bus Creator1 : BusCreator
  Cable length : Constant  Value=lL
  Gravity Constant : Constant  Value=g
  Mass Load : Constant  Value=mL
  Mass QR : Constant  Value=mQ
  Var : Outport
  wires:
  Mass QR/1 -> Bus Creator1/1  "mQ"
  Cable length/1 -> Bus Creator1/4  "lL"
  Mass Load/1 -> Bus Creator1/3  "mL"
  Bus Creator1/1 -> Var/1  "varddxL"
  Gravity Constant/1 -> Bus Creator1/2  "g"

== system QR2Dsim/QR-Load Subsystem/varQ ==
  Arm length : Constant  Value=l
  Bus Creator : BusCreator  Inputs=2
  Bus Creator1 : BusCreator  Inputs=8
  Cable length : Constant  Value=lL
  Drag Factor : Constant  Value=d
  Gravity Constant : Constant  Value=g
  Mass QR : Constant  Value=mQ
  QR Inertia : Constant  Value=diag([Ixx,Iyy,Izz])
  Rotor Inertia : Constant  Value=Ir
  Thrust Factor : Constant  Value=b
  ctauf : Constant  Value=ctauf
      mask Display: disp('c_{\tau f}','texmode','on')
  Var : Outport
  wires:
  Gravity Constant/1 -> Bus Creator/2  "g"
  Bus Creator/1 -> Var/1  "varQ"
  Mass QR/1 -> Bus Creator1/1  "m"
  Arm length/1 -> Bus Creator1/6  "l"
  Rotor Inertia/1 -> Bus Creator1/5  "Ir"
  QR Inertia/1 -> Bus Creator1/2  "I"
  Bus Creator1/1 -> Bus Creator/1  "sysvar"
  Thrust Factor/1 -> Bus Creator1/3  "b"
  Drag Factor/1 -> Bus Creator1/4  "d"
  ctauf/1 -> Bus Creator1/7  "ctauf"
  Cable length/1 -> Bus Creator1/8  "lL"

== system QR2Dsim/Control/QRL Load Attitude Controller/Subsystem3 ==
  note: Attitude Controlled Flight Mode
  note: Position Controlled Flight Mode Lee2010c
  note: Attitude Control 1
      | Position Control 0
  In1 : Inport
  In2 : Inport  Port=2
  In3 : Inport  Port=3
  Display : Display  Commented=on
  Gain1 : Gain  Commented=on
  Gain5 : Gain  Commented=on
  Subsystem : Subsystem  Commented=on
  Subsystem1 : Subsystem  Commented=on
  Subsystem2 : Subsystem  Commented=on
  Switch : Switch  Commented=on  Criteria=u2 > Threshold  Threshold=0.5
  To Workspace : ToWorkspace  Commented=on  VariableName=Re3  SampleTime=-1  SaveFormat=Structure With Time
  "e3 " : Gain  Commented=on  Gain=e3  Multiplication=Matrix(u*K)
  mode : Constant  Commented=on  Value=mode  VectorParams1D=off
  scope fatt fpos1 : Scope  Commented=on  NumInputPorts=2
      settings: ShowLegends=on  YMin=-11000~-200  YMax=5000~150  SaveName=ScopeData25
  Out1 : Outport
  Out2 : Outport  Port=2
  wires:
  In3/1 -> "e3 "/1
  "e3 "/1 -> Subsystem/5(Re3), Subsystem2/5(Re3), To Workspace/1
  Subsystem/1(fatt) -> Gain5/1
  Gain5/1 -> Switch/1, scope fatt fpos1/1  "fatt"
  Subsystem2/2(fpos) -> Switch/3, scope fatt fpos1/2  "fpos"
  Subsystem2/1(b3c/d) -> Gain1/1
  Subsystem1/4(mQge3) -> Subsystem/4(mQge3), Subsystem2/4(mQge3)
  In2/1 -> Subsystem1/2(QRoutputs)
  Subsystem1/1(mQddx) -> Subsystem/1(mQddx), Subsystem2/1(mQddx)
  Subsystem1/3(kvev) -> Subsystem/3(kvev), Subsystem2/3(kvev)
  Subsystem1/2(kxex) -> Subsystem/2(kxex), Subsystem2/2(kxex)
  mode/1 -> Display/1, Switch/2
  Switch/1 -> Out1/1  "f"
  In1/1 -> Subsystem1/1(xd)
  Gain1/1 -> Out2/1  "b3c/d"

== system QR2Dsim/Control/QRL QR Attitude Controller/QRL QR Attitude Controller ==
  note: Non-linear Geometric Attitude Controller
  note: QRL Load Attitude Control 3
      | QRL QR Attitude Control 2
  b1d : Inport
  QRoutputs : Inport  Port=2
  b1d1 : Inport  Port=3
  Display1 : Display
  Switch1 : Switch  Criteria=u2 > Threshold  Threshold=2.5
  mode1 : Constant  Value=mode  VectorParams1D=off
  phiQd : Constant  Value=phiQd  VectorParams1D=off
  M NL : Outport
  wires:
  mode1/1 -> Display1/1, Switch1/2
  b1d1/1 -> Switch1/1  "phiQc"
  phiQd/1 -> Switch1/3  "phiQd"

== system QR2Dsim/Control/QRL QR Attitude Controller/Subsystem ==
  note: Attitude Control 1
      | Position Control 0
  note: Attitude Controlled Flight Mode
  note: Position Controlled Flight Mode
  In1 : Inport
  In2 : Inport  Port=2
  In3 : Inport  Port=3
  In4 : Inport  Port=4
  In5 : Inport  Port=5
  In6 : Inport  Port=6
  Display : Display  Commented=on
  M NL Lee2010 : Subsystem  Commented=on
  M NL Lee2010c : Subsystem  Commented=on
  M lin : Subsystem  Commented=on
      mask Display: disp('Linear\n Attitude Controller')
  Switch : Switch  Commented=on  Criteria=u2 > Threshold  Threshold=0.5
  Terminator : Terminator  Commented=on
  mode : Constant  Value=mode  VectorParams1D=off
  Out1 : Outport
  wires:
  M lin/1(M lin) -> Terminator/1  "M lin"
  mode/1 -> Display/1, Switch/2
  M NL Lee2010/1(M NL) -> Switch/1  "Matt"
  M NL Lee2010c/1(M NL) -> Switch/3  "Mpos"
  In2/1 -> M NL Lee2010/1(R), M NL Lee2010c/1(R)
  Switch/1 -> Out1/1
  In4/1 -> M NL Lee2010/3(b1d)
  In1/1 -> M lin/1(QRoutputs), M NL Lee2010c/4(QRoutputs), M NL Lee2010/4(QRoutputs)
  In3/1 -> M NL Lee2010/2(b3d)
  In6/1 -> M NL Lee2010c/3(b1d)
  In5/1 -> M NL Lee2010c/2(b3d)

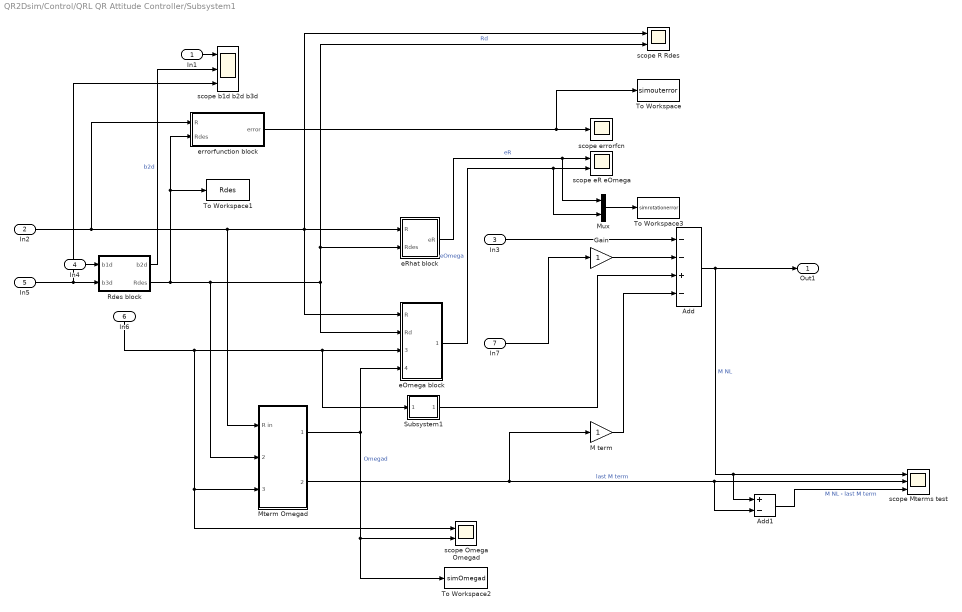
== system QR2Dsim/Control/QRL QR Attitude Controller/Subsystem1 ==
  In1 : Inport
  In2 : Inport  Port=2
  In3 : Inport  Port=3
  In4 : Inport  Port=4
  In5 : Inport  Port=5
  In6 : Inport  Port=6
  In7 : Inport  Port=7
  Add : Sum  Inputs=--+-
  Add1 : Sum  Inputs=+-
  Gain : Gain
  M term : Gain
  Mterm Omegad : Subsystem
  Mux : Mux  Inputs=2
  Rdes block : MATLAB Function  TreatAsAtomicUnit=on
  Subsystem1 : Subsystem
      mask Display: disp('\Omega \times I\Omega','texmode','on')
  To Workspace : ToWorkspace  VariableName=simouterror  SampleTime=-1  SaveFormat=Structure With Time
  To Workspace1 : ToWorkspace  VariableName=Rdes  SampleTime=-1  SaveFormat=Structure With Time
  To Workspace2 : ToWorkspace  VariableName=simOmegad  SampleTime=-1  SaveFormat=Structure With Time
  To Workspace3 : ToWorkspace  VariableName=simrotationerror  SampleTime=-1  SaveFormat=Structure With Time
  eOmega block : MATLAB Function  TreatAsAtomicUnit=on
  eRhat block : MATLAB Function  TreatAsAtomicUnit=on
  errorfunction block : MATLAB Function  TreatAsAtomicUnit=on
  scope Mterms test : Scope  NumInputPorts=3
      settings: YMin=-5~-5~-5  YMax=5~5~5  SaveName=ScopeData13
  scope Omega Omegad : Scope  NumInputPorts=2
      settings: ShowLegends=on  YMin=-5~-5  YMax=5~5  SaveName=scopeOmega
  scope R Rdes : Scope  NumInputPorts=2
      settings: ShowLegends=on  YMin=-5~-5  YMax=5~5  SaveName=ScopeData11
  scope b1d b2d b3d : Scope  NumInputPorts=3
      settings: ShowLegends=on  YMin=-5~-5~-5  YMax=5~5~5  SaveName=ScopeData10
  scope eR eOmega : Scope  NumInputPorts=2
      settings: YMin=-5~-5  YMax=5~5  SaveName=ScopeData8
  scope errorfcn : Scope
      settings: SaveName=scopeerrorfnc
  Out1 : Outport
  wires:
  Rdes block/1(b2d) -> scope b1d b2d b3d/2  "b2d"
  In2/1 -> eOmega block/1(R), scope R Rdes/1, eRhat block/1(R), Mterm Omegad/1(R in), errorfunction block/1(R)
  eRhat block/1(eR) -> Mux/1, scope eR eOmega/1  "eR"
  In3/1 -> Add/1
  In7/1 -> Gain/1
  eOmega block/1(eOmega) -> Mux/2, scope eR eOmega/2  "eOmega"
  In6/1 -> eOmega block/3(Omega), Subsystem1/1(Omega), scope Omega Omegad/1, Mterm Omegad/3(Omega in)
  Rdes block/2(Rdes) -> eOmega block/2(Rd), scope R Rdes/2, eRhat block/2(Rdes), Mterm Omegad/2(Rdes in), To Workspace1/1, errorfunction block/2(Rdes)  "Rd"
  Subsystem1/1(Out1) -> Add/3
  Add/1 -> Out1/1, Add1/1, scope Mterms test/1  "M NL"
  errorfunction block/1(error) -> To Workspace/1, scope errorfcn/1
  Mterm Omegad/2(M term) -> M term/1, Add1/2, scope Mterms test/2  "last M term"
  Mterm Omegad/1(Omegades) -> eOmega block/4(Omegad), To Workspace2/1, scope Omega Omegad/2  "Omegad"
  Gain/1 -> Add/2
  M term/1 -> Add/4
  Add1/1 -> scope Mterms test/3  "M NL - last M term"
  In5/1 -> scope b1d b2d b3d/3, Rdes block/2(b3d)
  Mux/1 -> To Workspace3/1
  In1/1 -> scope b1d b2d b3d/1
  In4/1 -> Rdes block/1(b1d)

== system QR2Dsim/QR Subsystem/dOmega block/Subsystem1 ==
  Omega : Inport
  Cross Product : vrlib/Utilities/Cross Product
  I : Gain  Gain=I  Multiplication=Matrix(K*u)
  Product1 : Product  Multiplication=Matrix(*)
  Terminator : Terminator
  fcnhat : MATLAB Function  TreatAsAtomicUnit=on
  Out1 : Outport
  wires:
  Omega/1 -> Cross Product/1, I/1, fcnhat/1(A)
  fcnhat/1(fcnhat) -> Product1/1
  I/1 -> Cross Product/2, Product1/2
  Cross Product/1 -> Out1/1
  Product1/1 -> Terminator/1

== system QR2Dsim/QR Subsystem/dOmega block/Subsystem2 ==
  In1 : Inport
  In2 : Inport  Port=2
  In3 : Inport  Port=3
  Constant : Constant  Value=e3
  Product : Product
  Product1 : Product  Multiplication=Matrix(*)
  Product2 : Product
  fcnhat1 : MATLAB Function  TreatAsAtomicUnit=on
  fcnomega : MATLAB Function  TreatAsAtomicUnit=on
  Out1 : Outport
  wires:
  Product2/1 -> Out1/1  "tau_G"
  In2/1 -> Product/1
  fcnomega/1(fcnomega) -> Product2/2
  Product1/1 -> Product/2
  In3/1 -> fcnomega/1(omega)
  In1/1 -> fcnhat1/1(A)
  fcnhat1/1(fcnhat) -> Product1/1
  Constant/1 -> Product1/2
  Product/1 -> Product2/1

== system QR2Dsim/QR-Load Subsystem/Integration Block/Initial dstates ==
  Bus Creator1 : BusCreator  Inputs=3
  OmegaL0 : Constant  Value=[pL0; qL0; rL0]
  OmegaQ0 : Constant  Value=[pQ0; qQ0; rQ0]
  dxL0 : Constant  Value=[dxL0;dyL0;dzL0]
  Init vel : Outport
  wires:
  dxL0/1 -> Bus Creator1/1  "dxL0"
  Bus Creator1/1 -> Init vel/1  "Init dstates"
  OmegaL0/1 -> Bus Creator1/2  "OmegaL0"
  OmegaQ0/1 -> Bus Creator1/3  "OmegaQ0"

== system QR2Dsim/QR-Load Subsystem/Integration Block/Initial states ==
  Bus Creator1 : BusCreator  Inputs=3
  angleL0 : Constant  Value=[phiL0; thetaL0; psiL0]
  angleQ0 : Constant  Value=[phiQ0; thetaQ0; psiQ0]
  xL0 : Constant  Value=[dxL0;dyL0;dzL0]
  Init vel : Outport
  wires:
  xL0/1 -> Bus Creator1/1  "xL0"
  Bus Creator1/1 -> Init vel/1  "Init states"
  angleL0/1 -> Bus Creator1/2  "angleL0"
  angleQ0/1 -> Bus Creator1/3  "angleQ0"

== system QR2Dsim/QR-Load Subsystem/dOmegaQ block/Subsystem1 ==
  Omega : Inport
  Cross Product : vrlib/Utilities/Cross Product
  I : Gain  Gain=I  Multiplication=Matrix(K*u)
  Product1 : Product  Multiplication=Matrix(*)
  Terminator : Terminator
  fcnhat : MATLAB Function  TreatAsAtomicUnit=on
  Out1 : Outport
  wires:
  Omega/1 -> Cross Product/1, I/1, fcnhat/1(A)
  fcnhat/1(fcnhat) -> Product1/1
  I/1 -> Cross Product/2, Product1/2
  Cross Product/1 -> Out1/1
  Product1/1 -> Terminator/1

== system QR2Dsim/QR-Load Subsystem/dOmegaQ block/Subsystem2 ==
  In1 : Inport
  In2 : Inport  Port=2
  In3 : Inport  Port=3
  Constant : Constant  Value=e3
  Product : Product
  Product1 : Product  Multiplication=Matrix(*)
  Product2 : Product
  fcnhat1 : MATLAB Function  TreatAsAtomicUnit=on
  fcnomega : MATLAB Function  TreatAsAtomicUnit=on
  Out1 : Outport
  wires:
  Product2/1 -> Out1/1  "tau_G"
  In2/1 -> Product/1
  fcnomega/1(fcnomega) -> Product2/2
  Product1/1 -> Product/2
  In3/1 -> fcnomega/1(omega)
  In1/1 -> fcnhat1/1(A)
  fcnhat1/1(fcnhat) -> Product1/1
  Constant/1 -> Product1/2
  Product/1 -> Product2/1

== system QR2Dsim/Control/QRL Load Attitude Controller/Subsystem3/Subsystem ==
  mQddx : Inport
  kxex : Inport  Port=2
  kvev : Inport  Port=3
  mQge3 : Inport  Port=4
  Re3 : Inport  Port=5
  Add : Sum  Inputs=+---
  Divide : Product  Inputs=*/
  Gain5 : Gain  Gain=-1
  Selector : Selector  InputPortWidth=3  IndexOptions=Index vector (dialog)  Indices=3  OutputSizes=1
  Selector1 : Selector  InputPortWidth=3  IndexOptions=Index vector (dialog)  Indices=3  OutputSizes=1
  fatt : Outport
  wires:
  Selector/1 -> Divide/1
  Selector1/1 -> Divide/2
  Add/1 -> Gain5/1
  Re3/1 -> Selector1/1
  mQge3/1 -> Add/4
  kxex/1 -> Add/2
  kvev/1 -> Add/3
  mQddx/1 -> Add/1
  Divide/1 -> fatt/1  "fatt"
  Gain5/1 -> Selector/1

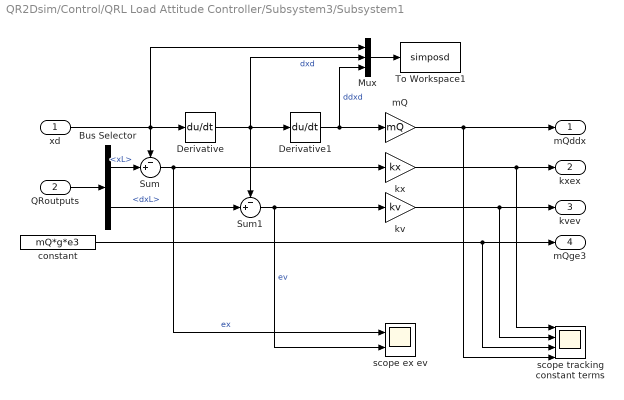
== system QR2Dsim/Control/QRL Load Attitude Controller/Subsystem3/Subsystem1 ==
  xd : Inport
  QRoutputs : Inport  Port=2
  Bus Selector : BusSelector  OutputSignals=xL,dxL
  Derivative : Derivative
  Derivative1 : Derivative
  Mux : Mux  Inputs=3
  Sum : Sum  Inputs=-+|
  Sum1 : Sum  Inputs=-+|
  To Workspace1 : ToWorkspace  VariableName=simposd  SampleTime=-1  SaveFormat=Structure With Time
  constant : Constant  Value=mQ*g*e3  VectorParams1D=off
  kv : Gain  Gain=kv
  kx : Gain  Gain=kx
  mQ : Gain  Gain=mQ
  scope ex ev : Scope  NumInputPorts=2
      settings: ShowLegends=on  YMin=-5~-5  YMax=5~5  SaveName=ScopeData7
  scope tracking constant terms : Scope  NumInputPorts=4
      settings: ShowLegends=on  YMin=-5~-5~-5~-5  YMax=5~5~5~5
  mQddx : Outport
  kxex : Outport  Port=2
  kvev : Outport  Port=3
  mQge3 : Outport  Port=4
  wires:
  xd/1 -> Mux/1, Derivative/1, Sum/1
  Derivative/1 -> Mux/2, Derivative1/1, Sum1/1  "dxd"
  Derivative1/1 -> Mux/3, mQ/1  "ddxd"
  QRoutputs/1 -> Bus Selector/1
  Bus Selector/1 -> Sum/2  "<xL>"
  Bus Selector/2 -> Sum1/2  "<dxL>"
  Sum1/1 -> kv/1, scope ex ev/2  "ev"
  Sum/1 -> kx/1, scope ex ev/1  "ex"
  kv/1 -> kvev/1, scope tracking constant terms/2
  constant/1 -> mQge3/1, scope tracking constant terms/3
  mQ/1 -> mQddx/1, scope tracking constant terms/4
  kx/1 -> kxex/1, scope tracking constant terms/1
  Mux/1 -> To Workspace1/1

== system QR2Dsim/Control/QRL Load Attitude Controller/Subsystem3/Subsystem2 ==
  mQddx : Inport
  kxex : Inport  Port=2
  kvev : Inport  Port=3
  mQge3 : Inport  Port=4
  Re3 : Inport  Port=5
  Add : Sum  Inputs=+---
  Dot Product : DotProduct  InputSameDT=on  OutDataTypeStr=Inherit: Inherit via internal rule
  Gain1 : Gain  Gain=-1
  Gain3 : Gain  Gain=-1
  Normalization : dspmathops/Normalization  NormType=2-norm  Bias=1e-10  NormOver=Each column  ColComp=on  Dimension=3  outputDataTypeStr=Inherit: Same as product output  outputLastDataTypeStr=Inherit: Same as product output  outputMin=[]  outputMax=[]  accumDataTypeStr=Inherit: Same as product output  accumLastDataTypeStr=Inherit: Same as product output  roundingMode=Floor  overflowMode=off
  Normalize Vector : vrlib/Utilities/Normalize Vector  maxzero=0
  scope b3c normal diff : Scope  NumInputPorts=2
      settings: ShowLegends=on  YMin=-5~-5  YMax=5~5  SaveName=ScopeData20
  scope tracking constant : Scope
      settings: ShowLegends=on  YMin=-10  YMax=10  SaveName=ScopeData18
  b3c/d : Outport
  fpos : Outport  Port=2
  wires:
  Normalize Vector/1 -> scope b3c normal diff/2
  Dot Product/1 -> fpos/1  "fpos"
  Add/1 -> Normalization/1, Normalize Vector/1, scope tracking constant/1, Gain1/1  "tracking constant"
  Normalization/1 -> Gain3/1, scope b3c normal diff/1
  Re3/1 -> Dot Product/2
  mQge3/1 -> Add/4
  kxex/1 -> Add/2
  kvev/1 -> Add/3
  mQddx/1 -> Add/1
  Gain3/1 -> b3c/d/1
  Gain1/1 -> Dot Product/1

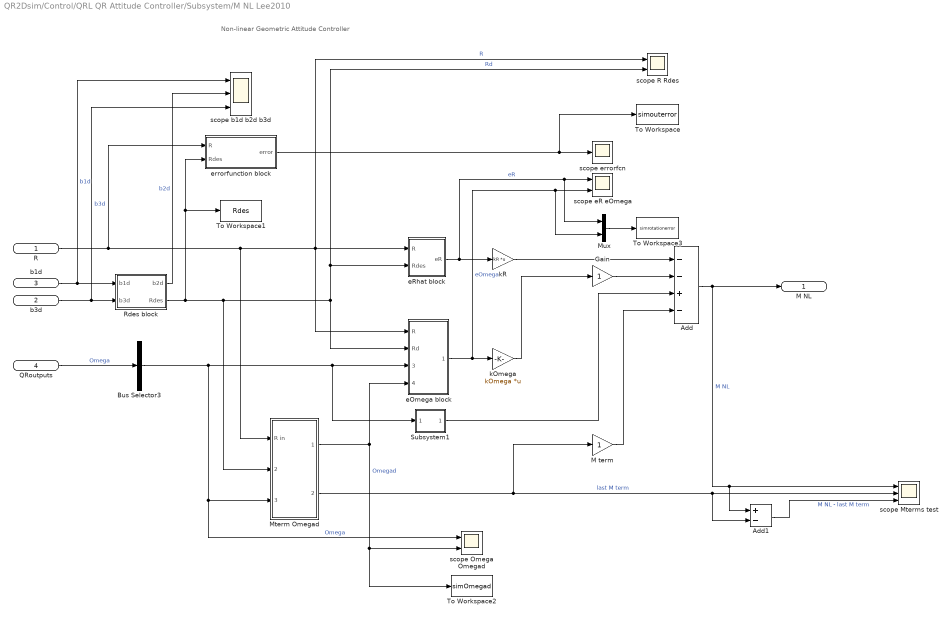
== system QR2Dsim/Control/QRL QR Attitude Controller/Subsystem/M NL Lee2010 ==
  note: Non-linear Geometric Attitude Controller
  R : Inport
  b3d : Inport  Port=2
  b1d : Inport  Port=3
  QRoutputs : Inport  Port=4
  Add : Sum  Inputs=--+-
  Add1 : Sum  Inputs=+-
  Bus Selector3 : BusSelector  OutputSignals=OmegaL  OutputAsBus=on
  Gain : Gain
  M term : Gain
  Mterm Omegad : Subsystem
  Mux : Mux  Inputs=2
  Rdes block : MATLAB Function  TreatAsAtomicUnit=on
  Subsystem1 : Subsystem
      mask Display: disp('\Omega \times I\Omega','texmode','on')
  To Workspace : ToWorkspace  VariableName=simouterror  SampleTime=-1  SaveFormat=Structure With Time
  To Workspace1 : ToWorkspace  VariableName=Rdes  SampleTime=-1  SaveFormat=Structure With Time
  To Workspace2 : ToWorkspace  VariableName=simOmegad  SampleTime=-1  SaveFormat=Structure With Time
  To Workspace3 : ToWorkspace  VariableName=simrotationerror  SampleTime=-1  SaveFormat=Structure With Time
  eOmega block : MATLAB Function  TreatAsAtomicUnit=on
  eRhat block : MATLAB Function  TreatAsAtomicUnit=on
  errorfunction block : MATLAB Function  TreatAsAtomicUnit=on
  kOmega : Gain  Gain=kOmega  Multiplication=Matrix(K*u)
  kR : Gain  Gain=kR  Multiplication=Matrix(K*u)
  scope Mterms test : Scope  NumInputPorts=3
      settings: YMin=-5~-5~-5  YMax=5~5~5  SaveName=ScopeData13
  scope Omega Omegad : Scope  NumInputPorts=2
      settings: ShowLegends=on  YMin=-5~-5  YMax=5~5  SaveName=scopeOmega
  scope R Rdes : Scope  NumInputPorts=2
      settings: ShowLegends=on  YMin=-5~-5  YMax=5~5  SaveName=ScopeData11
  scope b1d b2d b3d : Scope  NumInputPorts=3
      settings: ShowLegends=on  YMin=-5~-5~-5  YMax=5~5~5  SaveName=ScopeData10
  scope eR eOmega : Scope  NumInputPorts=2
      settings: YMin=-5~-5  YMax=5~5  SaveName=ScopeData8
  scope errorfcn : Scope
      settings: SaveName=scopeerrorfnc
  M NL : Outport
  wires:
  R/1 -> eOmega block/1(R), scope R Rdes/1, eRhat block/1(R), Mterm Omegad/1(R in), errorfunction block/1(R)  "R"
  eRhat block/1(eR) -> Mux/1, scope eR eOmega/1, kR/1  "eR"
  kR/1 -> Add/1
  kOmega/1 -> Gain/1
  eOmega block/1(eOmega) -> Mux/2, scope eR eOmega/2, kOmega/1  "eOmega"
  b1d/1 -> Rdes block/1(b1d), scope b1d b2d b3d/1  "b1d"
  QRoutputs/1 -> Bus Selector3/1  "Omega"
  Bus Selector3/1 -> eOmega block/3(Omega), Subsystem1/1(Omega), scope Omega Omegad/1, Mterm Omegad/3(Omega in)  "Omega"
  Rdes block/2(Rdes) -> eOmega block/2(Rd), scope R Rdes/2, eRhat block/2(Rdes), Mterm Omegad/2(Rdes in), To Workspace1/1, errorfunction block/2(Rdes)  "Rd"
  Rdes block/1(b2d) -> scope b1d b2d b3d/2  "b2d"
  Subsystem1/1(Out1) -> Add/3
  Add/1 -> Add1/1, scope Mterms test/1, M NL/1  "M NL"
  errorfunction block/1(error) -> To Workspace/1, scope errorfcn/1
  Mterm Omegad/2(M term) -> M term/1, Add1/2, scope Mterms test/2  "last M term"
  Mterm Omegad/1(Omegades) -> eOmega block/4(Omegad), To Workspace2/1, scope Omega Omegad/2  "Omegad"
  Gain/1 -> Add/2
  M term/1 -> Add/4
  Add1/1 -> scope Mterms test/3  "M NL - last M term"
  b3d/1 -> scope b1d b2d b3d/3, Rdes block/2(b3d)  "b3d"
  Mux/1 -> To Workspace3/1
